simulink model "simulator"  (R2021b)
settings: Solver=VariableStepAuto  StartTime=0.0  StopTime=10.0  RelTol=1e-3
libraries: shared6dof x1
settings Model: Creator=zhongyuliang  LastModifiedBy=zhongyuliang

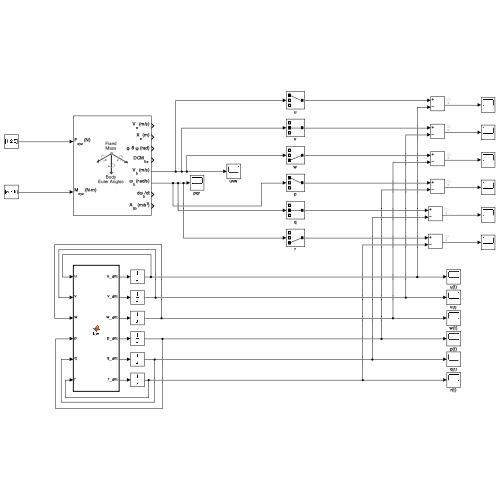
[thumbnail: Simulink's stored preview of the top-level diagram]
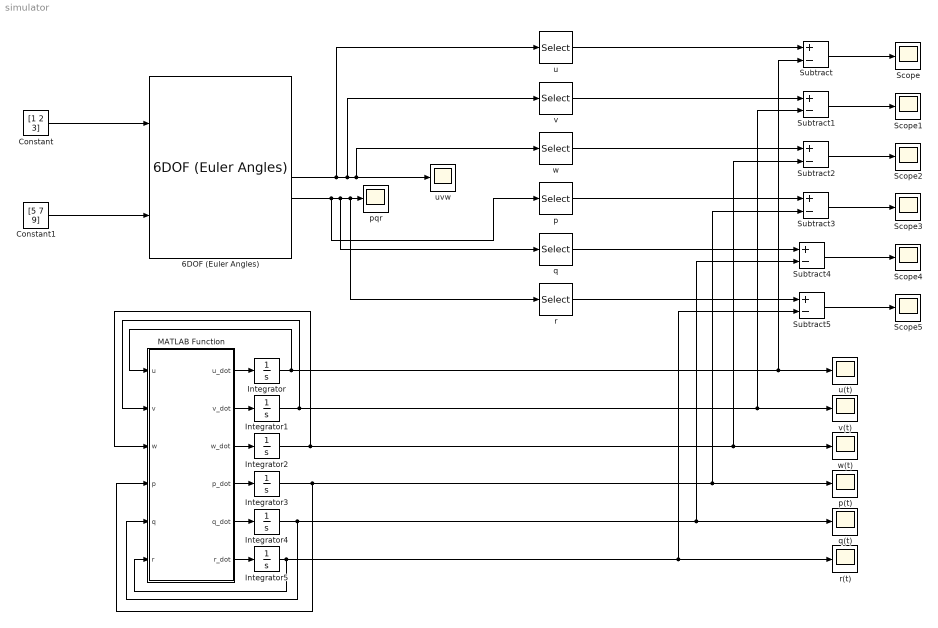
== system simulator ==
  6DOF (Euler Angles) : shared6dof/6DOF (Euler Angles)  units=Metric (MKS)  mtype=Fixed  rep=Euler Angles  xme_0=[0 0 0]  Vm_0=[0 0 0]  eul_0=[0 0 0]  pm_0=[0 0 0]  mass_0=1  mass_e=0.5  mass_f=2.0  inertia=|  inertia_e=eye(3)  inertia_f=2*eye(3)  k_quat=1.0  vre_flag=on  abi_flag=off  aMode=0  xme_statename=''  Vm_statename=''  eul_statename=''  quat_statename=''  pm_statename=''  mass_statename=''
      | [3.14, 2.17, 1.58;
      |          2.17, 5.12 ,6.44;
      |          1.58 ,6.44 ,9.75]
      settings: SourceProductBaseCode=AE,PW,DR,MT,UV,VE
  Constant : Constant  Value=[1 2 3]
  Constant1 : Constant  Value=[5 7 9]
  Integrator{,1..5} (6 alike) : Integrator
  MATLAB Function : MATLAB Function  TreatAsAtomicUnit=on
  Scope{,1..5} (6 alike) : Scope
  Subtract{,1..5} (6 alike) : Sum  Inputs=+-
  p : Selector  InputPortWidth=3  IndexOptions=Index vector (dialog)  Indices=1  OutputSizes=1
  p(t) : Scope
  pqr : Scope
  q : Selector  InputPortWidth=3  IndexOptions=Index vector (dialog)  Indices=2  OutputSizes=1
  q(t) : Scope
  r : Selector  InputPortWidth=3  IndexOptions=Index vector (dialog)  Indices=3  OutputSizes=1
  r(t) : Scope
  u : Selector  InputPortWidth=3  IndexOptions=Index vector (dialog)  Indices=1  OutputSizes=1
  u(t) : Scope
  uvw : Scope
  v : Selector  InputPortWidth=3  IndexOptions=Index vector (dialog)  Indices=2  OutputSizes=1
  v(t) : Scope
  w : Selector  InputPortWidth=3  IndexOptions=Index vector (dialog)  Indices=3  OutputSizes=1
  w(t) : Scope
  wires:
  MATLAB Function/1(u_dot) -> Integrator/1
  MATLAB Function/2(v_dot) -> Integrator1/1
  MATLAB Function/4(p_dot) -> Integrator3/1
  MATLAB Function/6(r_dot) -> Integrator5/1
  MATLAB Function/5(q_dot) -> Integrator4/1
  MATLAB Function/3(w_dot) -> Integrator2/1
  Integrator1/1 -> Subtract1/2, v(t)/1, MATLAB Function/2(v)
  Integrator2/1 -> MATLAB Function/3(w), Subtract2/2, w(t)/1
  Integrator5/1 -> MATLAB Function/6(r), Subtract5/2, r(t)/1
  Integrator4/1 -> MATLAB Function/5(q), Subtract4/2, q(t)/1
  Constant/1 -> 6DOF (Euler Angles)/1
  6DOF (Euler Angles)/5 -> u/1, v/1, uvw/1, w/1
  6DOF (Euler Angles)/6 -> p/1, q/1, r/1, pqr/1
  Integrator/1 -> MATLAB Function/1(u), Subtract/2, u(t)/1
  Integrator3/1 -> MATLAB Function/4(p), Subtract3/2, p(t)/1
  Constant1/1 -> 6DOF (Euler Angles)/2
  u/1 -> Subtract/1
  r/1 -> Subtract5/1
  q/1 -> Subtract4/1
  p/1 -> Subtract3/1
  w/1 -> Subtract2/1
  v/1 -> Subtract1/1
  Subtract/1 -> Scope/1
  Subtract1/1 -> Scope1/1
  Subtract2/1 -> Scope2/1
  Subtract3/1 -> Scope3/1
  Subtract4/1 -> Scope4/1
  Subtract5/1 -> Scope5/1

== matlab function simulator/MATLAB Function ==
  data: u input; u_dot output; v input; w input; p input; q input; r input; v_dot output; w_dot output; p_dot output; q_dot output; r_dot output
function [u_dot, v_dot, w_dot, p_dot, q_dot, r_dot] = fcn(u,v,w,p,q,r)
    B_F = [1;2;3];
    m = 1;
    B_M = [5;7;9];
    I = [3.14, 2.17, 1.58;
         2.17, 5.12 ,6.44;
         1.58 ,6.44 ,9.75];
%     I = eye(3);

    uvw = -skew([p;q;r;])*[u;v;w;] + B_F/m;
    u_dot = uvw(1);
    v_dot = uvw(2);
    w_dot = uvw(3);

    pqr = I\(B_M - skew([p;q;r])*I*[p;q;r]);
    p_dot = pqr(1);
    q_dot = pqr(2);
    r_dot = pqr(3);
end

function M = skew(a)
    M = [0,     -a(3), a(2);
         a(3),  0    , -a(1);
         -a(2), a(1) , 0];
end
